simulink model "SDOF_SMD"  (R2016a)
settings: Solver=VariableStepAuto  StartTime=0.0  StopTime=10.0  RelTol=1e-3
undefined symbols (not defined in the file): C, K, M
settings Model: Creator=ROB  LastModifiedBy=ROB

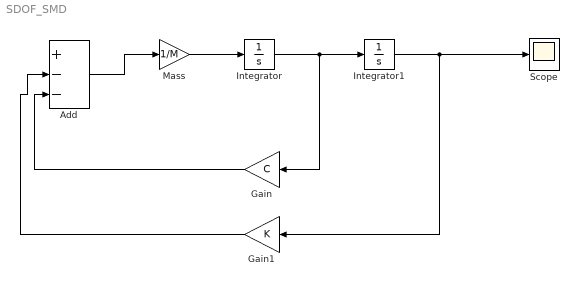
== system SDOF_SMD ==
  Add : Sum  Inputs=+--
  Gain : Gain  Gain=C
  Gain1 : Gain  Gain=K
  Integrator : Integrator
  Integrator1 : Integrator  InitialCondition=1
  Mass : Gain  Gain=1/M
  Scope : Scope
  wires:
  Add/1 -> Mass/1
  Mass/1 -> Integrator/1
  Integrator/1 -> Gain/1, Integrator1/1
  Gain/1 -> Add/3
  Integrator1/1 -> Gain1/1, Scope/1
  Gain1/1 -> Add/2
